simulink model "ans4_65070121_155_168"  (R2024b)
settings: Solver=VariableStepAuto  StartTime=0.0  StopTime=5  RelTol=1e-3
settings Model: Creator=picha  LastModifiedBy=picha

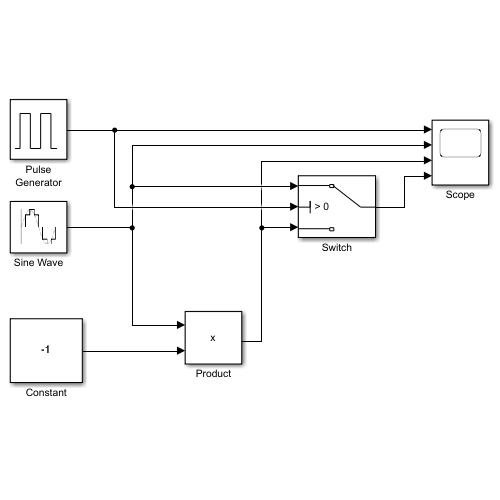
[thumbnail: Simulink's stored preview of the top-level diagram]
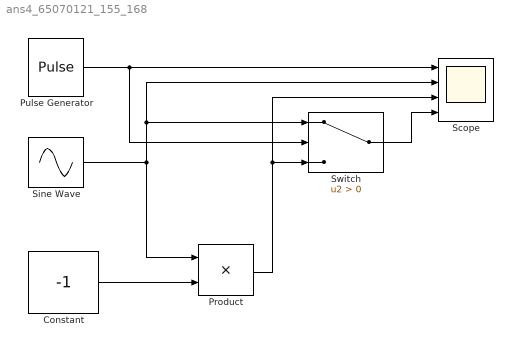
== system ans4_65070121_155_168 ==
  Constant : Constant  Value=-1
  Product : Product
  Pulse Generator : DiscretePulseGenerator  PulseType=Time based  PulseWidth=50
  Scope : Scope  NumInputPorts=4
  Sine Wave : Sin  Frequency=4*pi  SampleTime=0.001
  Switch : Switch  Criteria=u2 > Threshold  SaturateOnIntegerOverflow=off  InputSameDT=off
  wires:
  Pulse Generator/1 -> Switch/2, Scope/1
  Constant/1 -> Product/2
  Sine Wave/1 -> Product/1, Scope/2, Switch/1
  Product/1 -> Scope/3, Switch/3
  Switch/1 -> Scope/4
